simulink model "BPM_Compressor_Reciprocating"  (R2018a)
settings: Solver=FixedStepDiscrete  StartTime=0.0  StopTime=10.0  FixedStep=TimeSteps.ModelStep  RelTol=1e-3
InitFcn:
  | temp_script_1
libraries: FMIKit_blocks x1
settings Model: Creator=KIRTACA  LastModifiedBy=BEDNASA
settings SFSimCC: SimUserSources="\"C:\\Data\\Nucleus_Dev\\MCU_Sim_Arch_dev\\tools\\FMIKit_for_Simulink\\src\\FMU.cpp\" \"C:\\Data\\Nucleus_Dev\\MCU_Sim_Arch_dev\\tools\\FMIKit_for_Simulink\\src\\FMU1.cpp\" \"C:\\Data\\Nucleus_Dev\\MCU_Sim_Arch_dev\\tools\\FMIKit_for_Simulink\\src\\FMU2.cpp\" \"C:\\Data\\Nucleus_Dev\\MCU_Sim_Arch_2018\\tools\\FMIKit_for_Simulink\\src\\FMU.cpp\" \"C:\\Data\\Nucleus_Dev\\MCU_Sim_Arch_2018\\tools\\FMIKit_for_Simulink\\src\\FMU1.cpp\" \"C:\\Data\\Nucleus_Dev\\MCU_Sim_Arch_2018\\tools\\FMIKit_for_Simulink\\src\\FMU2.cpp\" \"C:\\Data\\Nucleus_Dev\\MCU_Sim_Arch_New_RotLoss\\tools\\FMIKit_for_Simulink\\src\\FMU.cpp\" \"C:\\Data\\Nucleus_Dev\\MCU_Sim_Arch_New_RotLoss\\tools\\FMIKit_for_Simulink\\src\\FMU1.cpp\" \"C:\\Data\\Nucleus_Dev\\MCU_Sim_Arch_New_RotLoss\\tools\\FMIKit_for_Simulink\\src\\FMU2.cpp\" \"C:\\Data\\Nucleus_Dev\\MCU_Sim_Arch_New_RotLoss_Test\\tools\\FMIKit_for_Simulink\\src\\FMU.cpp\" \"C:\\Data\\Nucleus_Dev\\MCU_Sim_Arch_New_RotLoss_Test\\tools\\FMIKit_for_Simulink\\src\\FMU1.cpp\" \"C:\\Data\\Nucleus_Dev\\MCU_Sim_Arch_New_RotLoss_Test\\tools\\FMIKit_for_Simulink\\src\\FMU2.cpp\" \"C:\\Data\\Nucleus_Dev\\MCU_Sim_Arch\\tools\\FMIKit_for_Simulink\\src\\FMU.cpp\" \"C:\\Data\\Nucleus_Dev\\MCU_Sim_Arch\\tools\\FMIKit_for_Simulink\\src\\FMU1.cpp\" \"C:\\Data\\Nucleus_Dev\\MCU_Sim_Arch\\tools\\FMIKit_for_Simulink\\src\\FMU2.cpp\""  SimUserIncludeDirs="\"C:\\Data\\Nucleus_Dev\\MCU_Sim_Arch_dev\\tools\\FMIKit_for_Simulink\\include\" \"C:\\Data\\Nucleus_Dev\\MCU_Sim_Arch_2018\\tools\\FMIKit_for_Simulink\\include\" \"C:\\Data\\Nucleus_Dev\\MCU_Sim_Arch_New_RotLoss\\tools\\FMIKit_for_Simulink\\include\" \"C:\\Data\\Nucleus_Dev\\MCU_Sim_Arch_New_RotLoss_Test\\tools\\FMIKit_for_Simulink\\include\" \"C:\\Data\\Nucleus_Dev\\MCU_Sim_Arch\\tools\\FMIKit_for_Simulink\\include\""
settings RTWCC: CustomInclude="\"C:\\Data\\Nucleus_Dev\\MCU_Sim_Arch_dev\\tools\\FMIKit_for_Simulink\\include\" \"C:\\Data\\Nucleus_Dev\\MCU_Sim_Arch_2018\\tools\\FMIKit_for_Simulink\\include\" \"C:\\Data\\Nucleus_Dev\\MCU_Sim_Arch_New_RotLoss\\tools\\FMIKit_for_Simulink\\include\" \"C:\\Data\\Nucleus_Dev\\MCU_Sim_Arch_New_RotLoss_Test\\tools\\FMIKit_for_Simulink\\include\" \"C:\\Data\\Nucleus_Dev\\MCU_Sim_Arch\\tools\\FMIKit_for_Simulink\\include\""  CustomSource="\"C:\\Data\\Nucleus_Dev\\MCU_Sim_Arch_dev\\tools\\FMIKit_for_Simulink\\src\\FMU.cpp\" \"C:\\Data\\Nucleus_Dev\\MCU_Sim_Arch_dev\\tools\\FMIKit_for_Simulink\\src\\FMU1.cpp\" \"C:\\Data\\Nucleus_Dev\\MCU_Sim_Arch_dev\\tools\\FMIKit_for_Simulink\\src\\FMU2.cpp\" \"C:\\Data\\Nucleus_Dev\\MCU_Sim_Arch_2018\\tools\\FMIKit_for_Simulink\\src\\FMU.cpp\" \"C:\\Data\\Nucleus_Dev\\MCU_Sim_Arch_2018\\tools\\FMIKit_for_Simulink\\src\\FMU1.cpp\" \"C:\\Data\\Nucleus_Dev\\MCU_Sim_Arch_2018\\tools\\FMIKit_for_Simulink\\src\\FMU2.cpp\" \"C:\\Data\\Nucleus_Dev\\MCU_Sim_Arch_New_RotLoss\\tools\\FMIKit_for_Simulink\\src\\FMU.cpp\" \"C:\\Data\\Nucleus_Dev\\MCU_Sim_Arch_New_RotLoss\\tools\\FMIKit_for_Simulink\\src\\FMU1.cpp\" \"C:\\Data\\Nucleus_Dev\\MCU_Sim_Arch_New_RotLoss\\tools\\FMIKit_for_Simulink\\src\\FMU2.cpp\" \"C:\\Data\\Nucleus_Dev\\MCU_Sim_Arch_New_RotLoss_Test\\tools\\FMIKit_for_Simulink\\src\\FMU.cpp\" \"C:\\Data\\Nucleus_Dev\\MCU_Sim_Arch_New_RotLoss_Test\\tools\\FMIKit_for_Simulink\\src\\FMU1.cpp\" \"C:\\Data\\Nucleus_Dev\\MCU_Sim_Arch_New_RotLoss_Test\\tools\\FMIKit_for_Simulink\\src\\FMU2.cpp\" \"C:\\Data\\Nucleus_Dev\\MCU_Sim_Arch\\tools\\FMIKit_for_Simulink\\src\\FMU.cpp\" \"C:\\Data\\Nucleus_Dev\\MCU_Sim_Arch\\tools\\FMIKit_for_Simulink\\src\\FMU1.cpp\" \"C:\\Data\\Nucleus_Dev\\MCU_Sim_Arch\\tools\\FMIKit_for_Simulink\\src\\FMU2.cpp\""
settings CodeAppCC: StateflowObjectComments=on

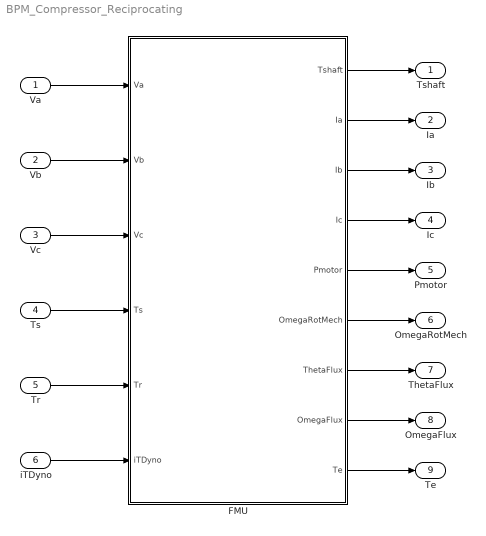
== system BPM_Compressor_Reciprocating ==
  Va : Inport
  Vb : Inport  Port=2
  Vc : Inport  Port=3
  Ts : Inport  Port=4
  Tr : Inport  Port=5
  iTDyno : Inport  Port=6
  FMU : Subsystem  Variant=on  VariantControl=Variant1
  Tshaft : Outport
  Ia : Outport  Port=2
  Ib : Outport  Port=3
  Ic : Outport  Port=4
  Pmotor : Outport  Port=5
  OmegaRotMech : Outport  Port=6
  ThetaFlux : Outport  Port=7
  OmegaFlux : Outport  Port=8
  Te : Outport  Port=9
  wires:
  Va/1 -> FMU/1("Va ")
  Vb/1 -> FMU/2("Vb ")
  Vc/1 -> FMU/3("Vc ")
  Ts/1 -> FMU/4("Ts ")
  Tr/1 -> FMU/5("Tr ")
  iTDyno/1 -> FMU/6("iTDyno ")
  FMU/1(" Tshaft") -> Tshaft/1
  FMU/2(" Ia") -> Ia/1
  FMU/3(" Ib") -> Ib/1
  FMU/4(" Ic") -> Ic/1
  FMU/5(" Pmotor") -> Pmotor/1
  FMU/6(" OmegaRotMech") -> OmegaRotMech/1
  FMU/7(" ThetaFlux") -> ThetaFlux/1
  FMU/8(" OmegaFlux") -> OmegaFlux/1
  FMU/9(" Te") -> Te/1

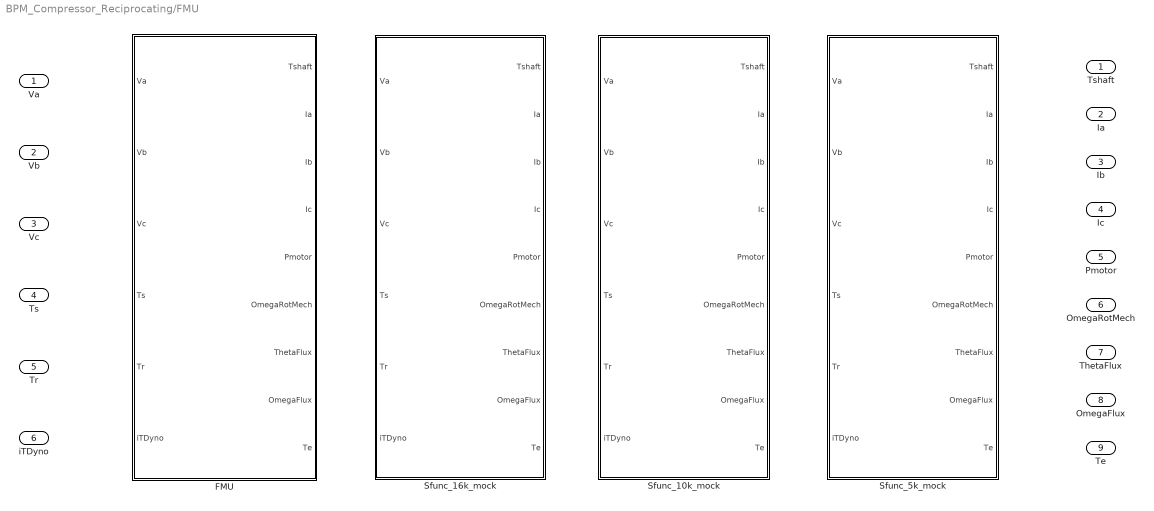
== system BPM_Compressor_Reciprocating/FMU ==
  "Va " : Inport
  "Vb " : Inport  Port=2
  "Vc " : Inport  Port=3
  "Ts " : Inport  Port=4
  "Tr " : Inport  Port=5
  "iTDyno " : Inport  Port=6
  FMU : Subsystem  VariantControl=Variant_Motor_Model_Executable == 1
  Sfunc_10k_mock : Subsystem  VariantControl=Variant_Motor_Model_Executable == 3
  Sfunc_16k_mock : Subsystem  VariantControl=Variant_Motor_Model_Executable == 2
  Sfunc_5k_mock : Subsystem  VariantControl=Variant_Motor_Model_Executable == 4
  " Tshaft" : Outport
  " Ia" : Outport  Port=2
  " Ib" : Outport  Port=3
  " Ic" : Outport  Port=4
  " Pmotor" : Outport  Port=5
  " OmegaRotMech" : Outport  Port=6
  " ThetaFlux" : Outport  Port=7
  " OmegaFlux" : Outport  Port=8
  " Te" : Outport  Port=9

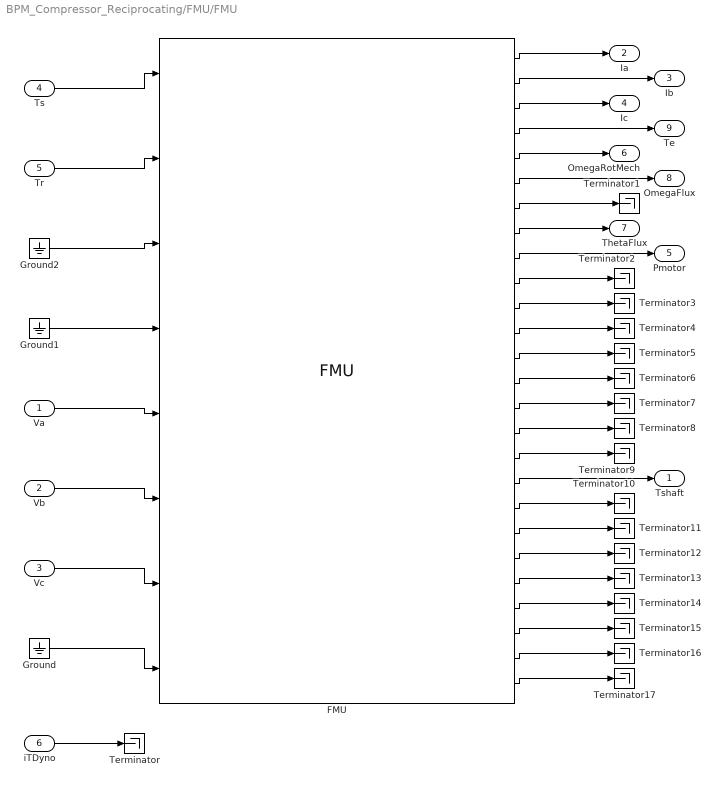
== system BPM_Compressor_Reciprocating/FMU/FMU ==
  Va : Inport
  Vb : Inport  Port=2
  Vc : Inport  Port=3
  Ts : Inport  Port=4
  Tr : Inport  Port=5
  iTDyno : Inport  Port=6
  FMU : FMIKit_blocks/FMU
      settings: SourceProductName=FMIKit
  Ground : Ground
  Ground1 : Ground
  Ground2 : Ground
  Terminator{,1..17} (18 alike) : Terminator
  Tshaft : Outport
  Ia : Outport  Port=2
  Ib : Outport  Port=3
  Ic : Outport  Port=4
  Pmotor : Outport  Port=5
  OmegaRotMech : Outport  Port=6
  ThetaFlux : Outport  Port=7
  OmegaFlux : Outport  Port=8
  Te : Outport  Port=9
  wires:
  Ts/1 -> FMU/1
  Tr/1 -> FMU/2
  Vc/1 -> FMU/7
  Vb/1 -> FMU/6
  Va/1 -> FMU/5
  iTDyno/1 -> Terminator/1
  Ground/1 -> FMU/8
  Ground1/1 -> FMU/4
  Ground2/1 -> FMU/3
  FMU/18 -> Tshaft/1
  FMU/9 -> Pmotor/1
  FMU/8 -> ThetaFlux/1
  FMU/6 -> OmegaFlux/1
  FMU/5 -> OmegaRotMech/1
  FMU/4 -> Te/1
  FMU/2 -> Ib/1
  FMU/1 -> Ia/1
  FMU/3 -> Ic/1
  FMU/7 -> Terminator1/1
  FMU/10 -> Terminator2/1
  FMU/11 -> Terminator3/1
  FMU/12 -> Terminator4/1
  FMU/13 -> Terminator5/1
  FMU/14 -> Terminator6/1
  FMU/15 -> Terminator7/1
  FMU/16 -> Terminator8/1
  FMU/17 -> Terminator9/1
  FMU/19 -> Terminator10/1
  FMU/20 -> Terminator11/1
  FMU/21 -> Terminator12/1
  FMU/22 -> Terminator13/1
  FMU/23 -> Terminator14/1
  FMU/24 -> Terminator15/1
  FMU/25 -> Terminator16/1
  FMU/26 -> Terminator17/1

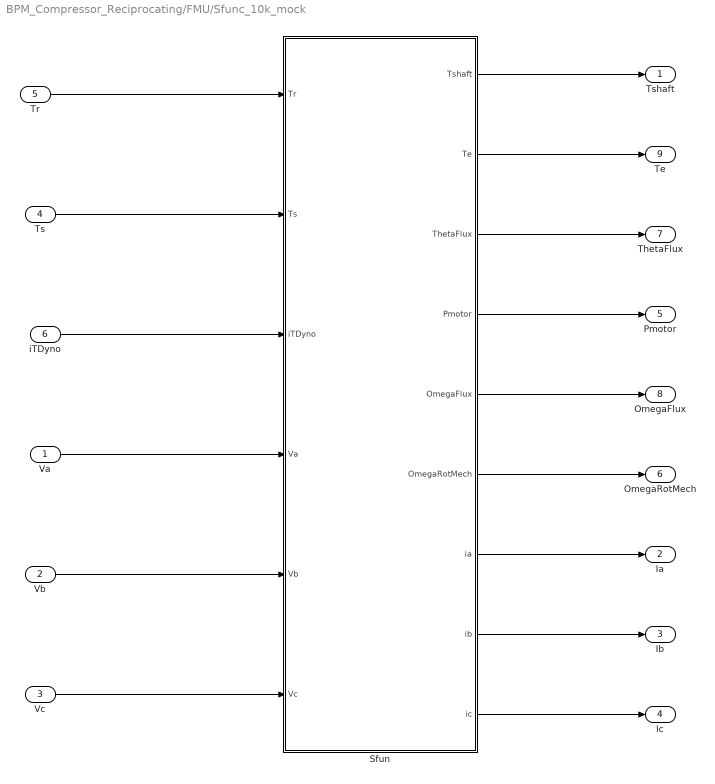
== system BPM_Compressor_Reciprocating/FMU/Sfunc_10k_mock ==
  Va : Inport
  Vb : Inport  Port=2
  Vc : Inport  Port=3
  Ts : Inport  Port=4
  Tr : Inport  Port=5
  iTDyno : Inport  Port=6
  Sfun : Subsystem  StartFcn=msgbox('Plant Model S-function is not available for this configuration. Please select the FMU Executable Variant in the GUI')
  Tshaft : Outport
  Ia : Outport  Port=2
  Ib : Outport  Port=3
  Ic : Outport  Port=4
  Pmotor : Outport  Port=5
  OmegaRotMech : Outport  Port=6
  ThetaFlux : Outport  Port=7
  OmegaFlux : Outport  Port=8
  Te : Outport  Port=9
  wires:
  Tr/1 -> Sfun/1(Tr)
  Ts/1 -> Sfun/2(Ts)
  Va/1 -> Sfun/4(Va)
  Vb/1 -> Sfun/5(Vb)
  Vc/1 -> Sfun/6(Vc)
  iTDyno/1 -> Sfun/3(iTDyno)
  Sfun/1(Tshaft) -> Tshaft/1
  Sfun/5(OmegaFlux) -> OmegaFlux/1
  Sfun/6(OmegaRotMech) -> OmegaRotMech/1
  Sfun/4(Pmotor) -> Pmotor/1
  Sfun/2(Te) -> Te/1
  Sfun/3(ThetaFlux) -> ThetaFlux/1
  Sfun/7(ia) -> Ia/1
  Sfun/8(ib) -> Ib/1
  Sfun/9(ic) -> Ic/1

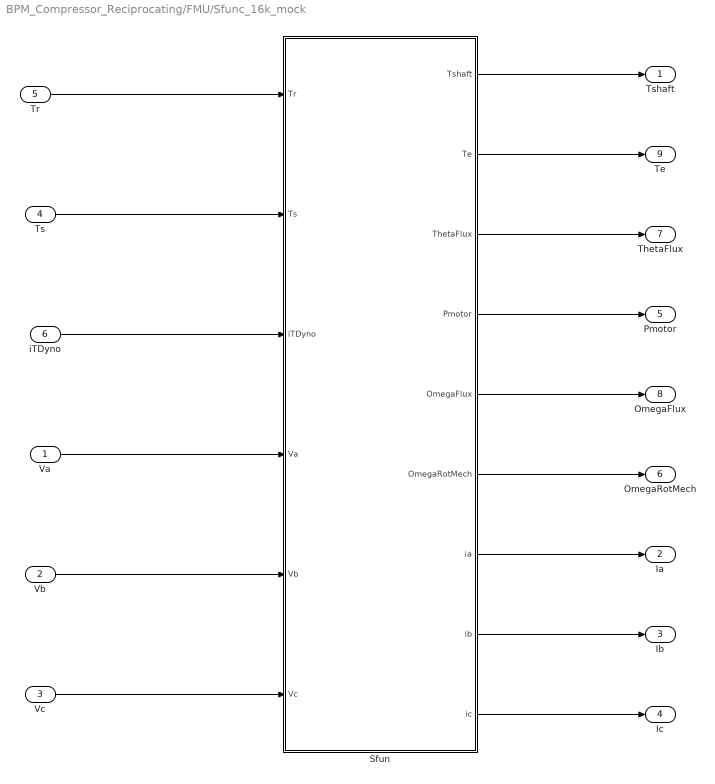
== system BPM_Compressor_Reciprocating/FMU/Sfunc_16k_mock ==
  Va : Inport
  Vb : Inport  Port=2
  Vc : Inport  Port=3
  Ts : Inport  Port=4
  Tr : Inport  Port=5
  iTDyno : Inport  Port=6
  Sfun : Subsystem  StartFcn=msgbox('Plant Model S-function is not available for this configuration. Please select the FMU Executable Variant in the GUI')
  Tshaft : Outport
  Ia : Outport  Port=2
  Ib : Outport  Port=3
  Ic : Outport  Port=4
  Pmotor : Outport  Port=5
  OmegaRotMech : Outport  Port=6
  ThetaFlux : Outport  Port=7
  OmegaFlux : Outport  Port=8
  Te : Outport  Port=9
  wires:
  Tr/1 -> Sfun/1(Tr)
  Ts/1 -> Sfun/2(Ts)
  Va/1 -> Sfun/4(Va)
  Vb/1 -> Sfun/5(Vb)
  Vc/1 -> Sfun/6(Vc)
  iTDyno/1 -> Sfun/3(iTDyno)
  Sfun/1(Tshaft) -> Tshaft/1
  Sfun/5(OmegaFlux) -> OmegaFlux/1
  Sfun/6(OmegaRotMech) -> OmegaRotMech/1
  Sfun/4(Pmotor) -> Pmotor/1
  Sfun/2(Te) -> Te/1
  Sfun/3(ThetaFlux) -> ThetaFlux/1
  Sfun/7(ia) -> Ia/1
  Sfun/8(ib) -> Ib/1
  Sfun/9(ic) -> Ic/1

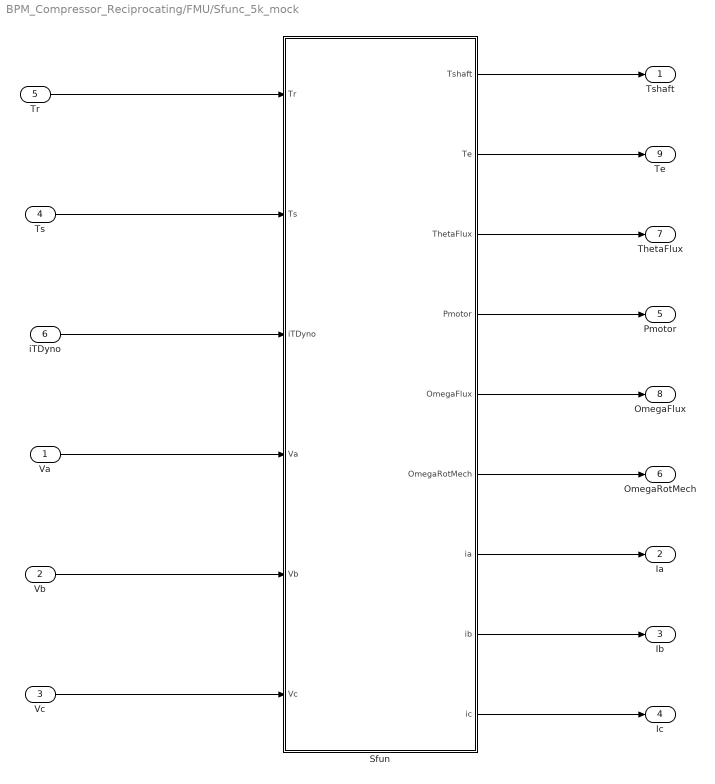
== system BPM_Compressor_Reciprocating/FMU/Sfunc_5k_mock ==
  Va : Inport
  Vb : Inport  Port=2
  Vc : Inport  Port=3
  Ts : Inport  Port=4
  Tr : Inport  Port=5
  iTDyno : Inport  Port=6
  Sfun : Subsystem  StartFcn=msgbox('Plant Model S-function is not available for this configuration. Please select the FMU Executable Variant in the GUI')
  Tshaft : Outport
  Ia : Outport  Port=2
  Ib : Outport  Port=3
  Ic : Outport  Port=4
  Pmotor : Outport  Port=5
  OmegaRotMech : Outport  Port=6
  ThetaFlux : Outport  Port=7
  OmegaFlux : Outport  Port=8
  Te : Outport  Port=9
  wires:
  Tr/1 -> Sfun/1(Tr)
  Ts/1 -> Sfun/2(Ts)
  Va/1 -> Sfun/4(Va)
  Vb/1 -> Sfun/5(Vb)
  Vc/1 -> Sfun/6(Vc)
  iTDyno/1 -> Sfun/3(iTDyno)
  Sfun/1(Tshaft) -> Tshaft/1
  Sfun/5(OmegaFlux) -> OmegaFlux/1
  Sfun/6(OmegaRotMech) -> OmegaRotMech/1
  Sfun/4(Pmotor) -> Pmotor/1
  Sfun/2(Te) -> Te/1
  Sfun/3(ThetaFlux) -> ThetaFlux/1
  Sfun/7(ia) -> Ia/1
  Sfun/8(ib) -> Ib/1
  Sfun/9(ic) -> Ic/1

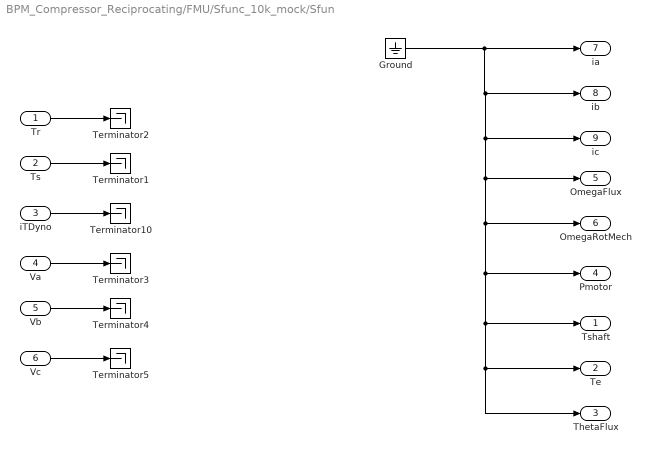
== system BPM_Compressor_Reciprocating/FMU/Sfunc_10k_mock/Sfun ==
  Tr : Inport
  Ts : Inport  Port=2
  iTDyno : Inport  Port=3
  Va : Inport  Port=4
  Vb : Inport  Port=5
  Vc : Inport  Port=6
  Ground : Ground
  Terminator{1..5,10} (6 alike) : Terminator
  Tshaft : Outport
  Te : Outport  Port=2
  ThetaFlux : Outport  Port=3
  Pmotor : Outport  Port=4
  OmegaFlux : Outport  Port=5
  OmegaRotMech : Outport  Port=6
  ia : Outport  Port=7
  ib : Outport  Port=8
  ic : Outport  Port=9
  wires:
  iTDyno/1 -> Terminator10/1
  Ts/1 -> Terminator1/1
  Tr/1 -> Terminator2/1
  Va/1 -> Terminator3/1
  Vb/1 -> Terminator4/1
  Vc/1 -> Terminator5/1
  Ground/1 -> OmegaRotMech/1, ThetaFlux/1, Te/1, Tshaft/1, Pmotor/1, OmegaFlux/1, ic/1, ib/1, ia/1

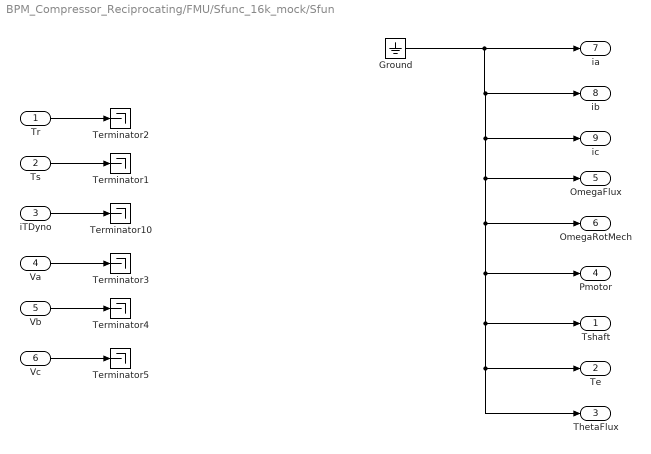
== system BPM_Compressor_Reciprocating/FMU/Sfunc_16k_mock/Sfun ==
  Tr : Inport
  Ts : Inport  Port=2
  iTDyno : Inport  Port=3
  Va : Inport  Port=4
  Vb : Inport  Port=5
  Vc : Inport  Port=6
  Ground : Ground
  Terminator{1..5,10} (6 alike) : Terminator
  Tshaft : Outport
  Te : Outport  Port=2
  ThetaFlux : Outport  Port=3
  Pmotor : Outport  Port=4
  OmegaFlux : Outport  Port=5
  OmegaRotMech : Outport  Port=6
  ia : Outport  Port=7
  ib : Outport  Port=8
  ic : Outport  Port=9
  wires:
  iTDyno/1 -> Terminator10/1
  Ts/1 -> Terminator1/1
  Tr/1 -> Terminator2/1
  Va/1 -> Terminator3/1
  Vb/1 -> Terminator4/1
  Vc/1 -> Terminator5/1
  Ground/1 -> OmegaRotMech/1, ThetaFlux/1, Te/1, Tshaft/1, Pmotor/1, OmegaFlux/1, ic/1, ib/1, ia/1

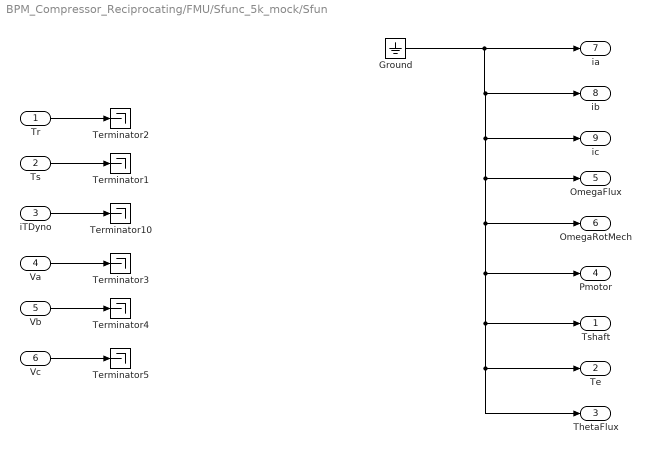
== system BPM_Compressor_Reciprocating/FMU/Sfunc_5k_mock/Sfun ==
  Tr : Inport
  Ts : Inport  Port=2
  iTDyno : Inport  Port=3
  Va : Inport  Port=4
  Vb : Inport  Port=5
  Vc : Inport  Port=6
  Ground : Ground
  Terminator{1..5,10} (6 alike) : Terminator
  Tshaft : Outport
  Te : Outport  Port=2
  ThetaFlux : Outport  Port=3
  Pmotor : Outport  Port=4
  OmegaFlux : Outport  Port=5
  OmegaRotMech : Outport  Port=6
  ia : Outport  Port=7
  ib : Outport  Port=8
  ic : Outport  Port=9
  wires:
  iTDyno/1 -> Terminator10/1
  Ts/1 -> Terminator1/1
  Tr/1 -> Terminator2/1
  Va/1 -> Terminator3/1
  Vb/1 -> Terminator4/1
  Vc/1 -> Terminator5/1
  Ground/1 -> OmegaRotMech/1, ThetaFlux/1, Te/1, Tshaft/1, Pmotor/1, OmegaFlux/1, ic/1, ib/1, ia/1
